simulink model "SRM_Circ_control"  (R2020a)
settings: Solver=VariableStepAuto  StartTime=0.0  StopTime=2  RelTol=1e-3
undefined symbols (not defined in the file): DiscIntNeverNeededParam, Ts
libraries: powerlib x18, powerlib_meascontrol x1
settings Model: Creator=NIKHIL  LastModifiedBy=NIKHIL

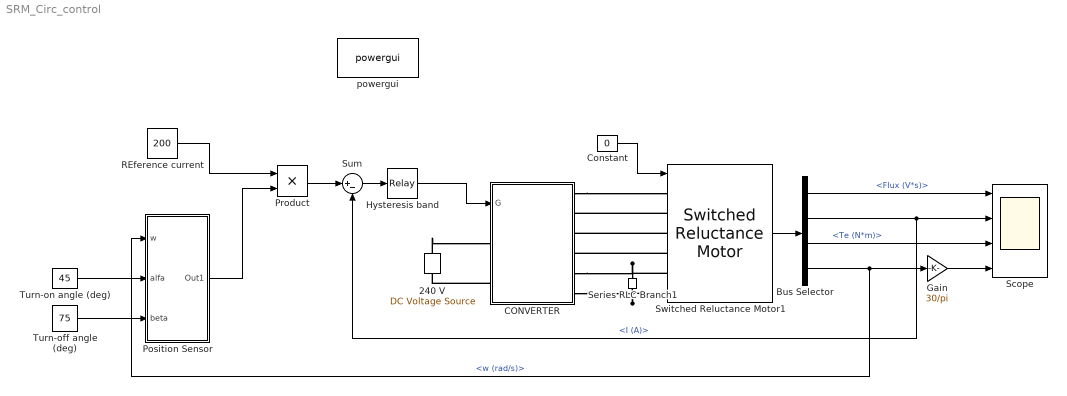
== system SRM_Circ_control ==
  240 V : powerlib/Electrical Sources/DC Voltage Source  Amplitude=240  Measurements=None
  Bus Selector : BusSelector  OutputSignals=Flux (V*s),I (A),Te (N*m),w (rad/s)
  CONVERTER : Subsystem
  Constant : Constant  Value=0
  Gain : Gain  Gain=30/pi
  "Hysteresis band " : Relay  OnSwitchValue=10  OffSwitchValue=-10
  Position Sensor : Subsystem
  Product : Product
  REference current : Constant  Value=200
  Scope : Scope  NumInputPorts=4
  Series RLC Branch1 : powerlib/Elements/Series RLC Branch  LConnTagsString=__new0  RConnTagsString=__new0  BranchType=R  Resistance=0.1  Inductance=1e-3  SetiL0=off  InitialCurrent=0  Capacitance=1e-6  Setx0=off  InitialVoltage=0  Measurements=None
  Sum : Sum  Inputs=|+-
  Switched Reluctance Motor1 : powerlib/Machines/Switched Reluctance Motor  MachineType=6/4  StatorResistance=0.05  Inertia=0.05  Friction=0.02  InitialSpeed=[0 0]  TsPowergui=0  TsBlock=Ts  MachineModel=Specific model  Lq=0.67e-3  Ld=23.6e-3  Lsat=0.15e-3  MaximumCurrent=450  MaximumFluxLinkage=0.486  Source=MAT-file  MagnetisationCharacteristic='srm64_60kw.mat'  RotorAngleVector=[0 10 20 30 40 45]  StatorCurrentVector=[0:25:450]  PlotCurves=off
      settings: SourceProductBaseCode=PS
  "Turn-off angle (deg) " : Constant  Value=75
  "Turn-on angle (deg) " : Constant  Value=45
  powergui : powerlib/powergui  Priority=1  SimulationMode=Discrete  SampleTime=1e-06  frequency=60  Iterations=50  frequencyindice=0  Pbase=100e6  ErrMax=1e-4  UnitsV=kV  UnitsW=MW  buscounter=0  FunctionMessages=off  echomessages=off  EnableUseOfTLC=off  CurrentSourceSwitches=off  DisableSnubberDevices=off  DisableRonSwitches=off  DisableVfSwitches=off  DisplayEquations=off  AutomaticDiscreteSolvers=off  SolverType=Tustin/Backward Euler (TBE)  Interpol=off  ExternalGateDelay=off  methode=off  Ts=100  x0status=blocks  SPID=on  SwTol=0  HookPort=off  NonlinearTolerance=0  nMaxIteration=15  ContinueOnMaxIteration=off  RestoreLinks=warning  ResistiveCurrentMeasurement=off  Frange=[0:2:500]  Ylog=off  Xlog=on  ShowGrid=off  save=off  variable=ZData  structure=0  ZoomFFT=off  StartTime=0.0  cycles=1  DisplayStyle=1  fundamental=60  FreqAxis=off  MaxFrequency=1000  frequencyindicesteady=1  RmsSteady=1  display=off
  wires:
  Sum/1 -> "Hysteresis band "/1
  "Hysteresis band "/1 -> CONVERTER/1(G)
  "Turn-on angle (deg) "/1 -> Position Sensor/2(alfa)
  "Turn-off angle (deg) "/1 -> Position Sensor/3(beta)
  Switched Reluctance Motor1/1 -> Bus Selector/1
  Constant/1 -> Switched Reluctance Motor1/1
  Bus Selector/2 -> Sum/2, Scope/2  "<I (A)>"
  Bus Selector/4 -> Position Sensor/1(w), Gain/1  "<w (rad/s)>"
  Bus Selector/1 -> Scope/1  "<Flux (V*s)>"
  REference current/1 -> Product/1
  Position Sensor/1(Out1) -> Product/2
  Gain/1 -> Scope/4
  Product/1 -> Sum/1
  Bus Selector/3 -> Scope/3  "<Te (N*m)>"
  connections:
  Series RLC Branch1/RConn1 -- CONVERTER/RConn6 -- Switched Reluctance Motor1/LConn6
  Series RLC Branch1/LConn1 -- CONVERTER/RConn5 -- Switched Reluctance Motor1/LConn5
  CONVERTER/RConn1 -- Switched Reluctance Motor1/LConn1
  Switched Reluctance Motor1/LConn3 -- CONVERTER/RConn3
  Switched Reluctance Motor1/LConn2 -- CONVERTER/RConn2
  Switched Reluctance Motor1/LConn4 -- CONVERTER/RConn4
  240 V/RConn1 -- CONVERTER/LConn1
  CONVERTER/LConn2 -- 240 V/LConn1

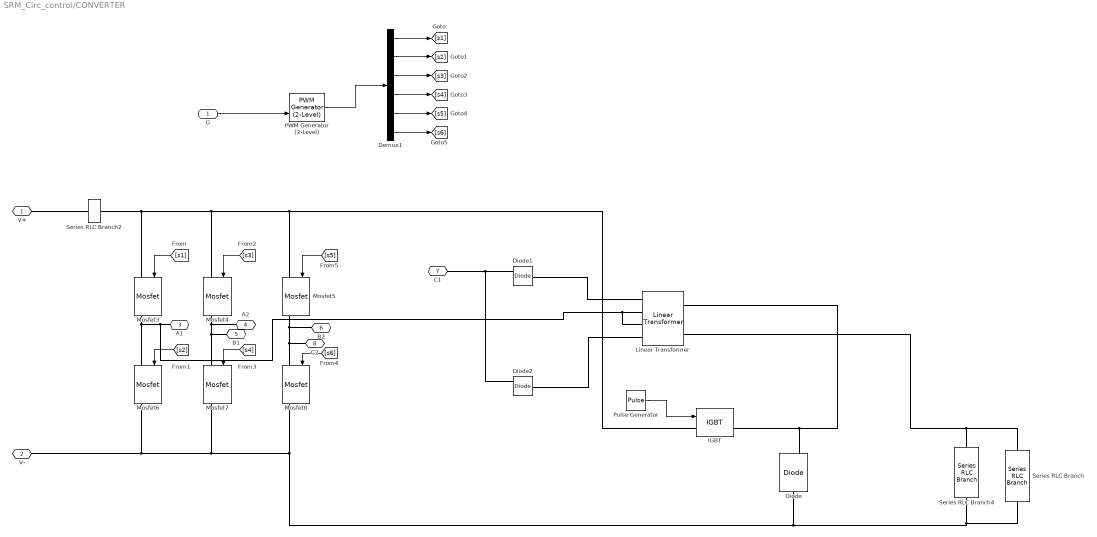
== system SRM_Circ_control/CONVERTER ==
  G : Inport
  Demux1 : Demux  Outputs=6
  Diode : powerlib/Power Electronics/Diode  Ron=0.001  Lon=0  Vf=0.8  IC=0  UseSnubber=0  Rs=500  Cs=250e-9  Measurements=on
  Diode1 : powerlib/Power Electronics/Diode  Ron=0.001  Lon=0  Vf=0.8  IC=0  UseSnubber=0  Rs=500  Cs=250e-9  Measurements=on
  Diode2 : powerlib/Power Electronics/Diode  Ron=0.001  Lon=0  Vf=0.8  IC=0  UseSnubber=0  Rs=500  Cs=250e-9  Measurements=on
  IGBT : powerlib/Power Electronics/IGBT  Ron=0.001  Lon=0  Vf=1  Tf=1e-6  Tt=2e-6  IC=0  Rs=1e5  Cs=inf  Measurements=on
  Linear Transformer : powerlib/Elements/Linear Transformer  UNITS=pu  NominalPower=[ 250e6 60 ]  winding1="[ 735e3  0.002  0.08 ]"  winding2="[ 315e3  0.002  0.08 ]"  ThreeWindings=on  winding3=[ 315e3 0.002 0.08 ]  RmLm=[ 500 500 ]  Measurements=None  DataType=off
  Mosfet{3..8} (6 alike) : powerlib/Power Electronics/Mosfet  Ron=0.1  Lon=0  Rd=0.01  Vfd=0  IC=0  Rs=1e5  Cs=inf  Measurements=on
  PWM Generator (2-Level) : powerlib_meascontrol/Pulse & Signal Generators/PWM Generator (2-Level)  ModulatorType=Three-phase bridge (6 pulses)  ModulatorMode=Synchronized  Fc=27*60  Pc=90  nF=27  MinMax="[ -1  1 ]"  SamplingTechnique=Natural  ModulatingSignals=off  m=0.8  Freq=60  Phase=0  Ts=0  ShowCarrierOutport=off
  Pulse Generator : DiscretePulseGenerator  PulseType=Time based  Period=1/10000  PulseWidth=50
  Series RLC Branch : powerlib/Elements/Series RLC Branch  LConnTagsString=__new0  RConnTagsString=__new0  BranchType=R  Resistance=1  Inductance=1e-3  SetiL0=off  InitialCurrent=0  Capacitance=1e-6  Setx0=off  InitialVoltage=0  Measurements=None
  Series RLC Branch2 : powerlib/Elements/Series RLC Branch  LConnTagsString=__new0  RConnTagsString=__new0  BranchType=R  Resistance=0.1  Inductance=1e-3  SetiL0=off  InitialCurrent=0  Capacitance=1e-6  Setx0=off  InitialVoltage=0  Measurements=None
  Series RLC Branch4 : powerlib/Elements/Series RLC Branch  LConnTagsString=__new0  RConnTagsString=__new0  BranchType=C  Resistance=1  Inductance=220e-3  SetiL0=off  InitialCurrent=0  Capacitance=220e-6  Setx0=off  InitialVoltage=0  Measurements=None
  V+ : PMIOPort  Side=Left
  V- : PMIOPort  Port=2  Side=Left
  A1 : PMIOPort  Port=3  Side=Right
  A2 : PMIOPort  Port=4  Side=Right
  B1 : PMIOPort  Port=5  Side=Right
  B2 : PMIOPort  Port=6  Side=Right
  C1 : PMIOPort  Port=7  Side=Right
  C2 : PMIOPort  Port=8  Side=Right
  wires:
  Demux1/6 -> [s6]
  Demux1/2 -> [s2]
  Demux1/1 -> [s1]
  Demux1/3 -> [s3]
  Demux1/5 -> [s5]
  Demux1/4 -> [s4]
  [s1] -> Mosfet3/1
  [s2] -> Mosfet6/1
  [s4] -> Mosfet7/1
  [s3] -> Mosfet4/1
  [s5] -> Mosfet5/1
  [s6] -> Mosfet8/1
  PWM Generator (2-Level)/1 -> Demux1/1
  G/1 -> PWM Generator (2-Level)/2
  Pulse Generator/1 -> IGBT/1
  connections:
  C2/RConn1 -- Mosfet8/LConn1 -- B2/RConn1 -- Mosfet5/RConn1
  Mosfet4/LConn1 -- Series RLC Branch2/RConn1 -- Mosfet3/LConn1 -- Mosfet5/LConn1 -- IGBT/LConn1
  Linear Transformer/RConn4 -- Diode2/LConn1
  Linear Transformer/RConn1 -- Diode1/LConn1
  Mosfet4/RConn1 -- A2/RConn1 -- B1/RConn1 -- Mosfet7/LConn1
  Mosfet8/RConn1 -- V-/RConn1 -- Mosfet6/RConn1 -- Mosfet7/RConn1 -- Series RLC Branch/RConn1 -- Series RLC Branch4/RConn1 -- Diode/LConn1
  Diode2/RConn1 -- C1/RConn1 -- Diode1/RConn1
  V+/RConn1 -- Series RLC Branch2/LConn1
  Mosfet3/RConn1 -- Linear Transformer/RConn3 -- Linear Transformer/RConn2 -- A1/RConn1 -- Mosfet6/LConn1
  Series RLC Branch4/LConn1 -- Series RLC Branch/LConn1 -- Linear Transformer/LConn2
  IGBT/RConn1 -- Linear Transformer/LConn1 -- Diode/RConn1

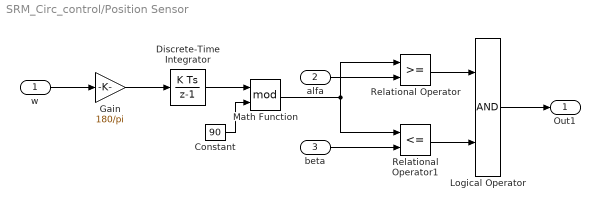
== system SRM_Circ_control/Position Sensor ==
  w : Inport
  alfa : Inport  Port=2
  beta : Inport  Port=3
  Constant : Constant  Value=90
  Discrete-Time Integrator : DiscreteIntegrator  InitialCondition=[0 -30 -60]  SampleTime=Ts  ICPrevOutput=DiscIntNeverNeededParam  ICPrevScaledInput=DiscIntNeverNeededParam
  Gain : Gain  Gain=180/pi
  Logical Operator : Logic  AllPortsSameDT=off  OutDataTypeStr=boolean
  Math Function : Math  Operator=mod  SignedPower=on  SaturateOnIntegerOverflow=on
  Relational Operator : RelationalOperator  OutDataTypeStr=boolean  RndMeth=Simplest
  Relational Operator1 : RelationalOperator  Operator=<=  OutDataTypeStr=boolean  RndMeth=Simplest
  Out1 : Outport  VectorParamsAs1DForOutWhenUnconnected=off
  wires:
  w/1 -> Gain/1
  Gain/1 -> Discrete-Time Integrator/1
  Discrete-Time Integrator/1 -> Math Function/1
  Constant/1 -> Math Function/2
  Math Function/1 -> Relational Operator/1, Relational Operator1/1
  alfa/1 -> Relational Operator/2
  beta/1 -> Relational Operator1/2
  Relational Operator/1 -> Logical Operator/1
  Relational Operator1/1 -> Logical Operator/2
  Logical Operator/1 -> Out1/1
